simulink model "CascadeControlSim"  (R2022b)
settings: Solver=VariableStepAuto  StartTime=0.0  StopTime=10.0  RelTol=1e-3
values from neighbouring files (symbols this model uses):
  biais_gyr = 1    [Set_Context_CFTE.m]
  Fmax = 0.17*PWM_max + -176.21    (= 121.29)    [Set_Context_CFTE.m]
  Fmin = 0.17*PWM_min + -176.21    (= 2.29)    [Set_Context_CFTE.m]
  Fmoy = 0.17*PWM_moy + -176.21    (= 53.29)    [Set_Context_CFTE.m]
  fr = 0.1    [Set_Context_CFTE.m]
  freq = 0.5    [Set_Context_CFTE.m]
  g = 9.81    [Set_Context_CFTE.m]
  I = 0.07110579    [Set_Context_CFTE.m]
  K1 = 4    [Set_Context_CFTE.m]
  K2 = 128    [Set_Context_CFTE.m]
  Kteta = 20    [Set_Context_CFTE.m]
  l1 = l2    (= 0.363)    [Set_Context_CFTE.m]
  sigma_acc = 0.022    [Set_Context_CFTE.m]
  sigma_gyr = 0.01047    [Set_Context_CFTE.m]
  Tcalibration = 0.5    [Set_Context_CFTE.m]
  Techelon = 4    [Set_Context_CFTE.m]
  theta_max = 0.785398    [Set_Context_CFTE.m]
  theta_ref = -pi()/4    [Set_Context_CFTE.m]
  Ts = 0.08    [Set_Context_CFTE.m]
undefined symbols (not defined in the file or in its folder): DiscIntNeverNeededParam, Rows
libraries: simulink x2, dspsigops x1, dspsrcs4 x1
settings Model: Creator=Hugo  LastModifiedBy=Hugo

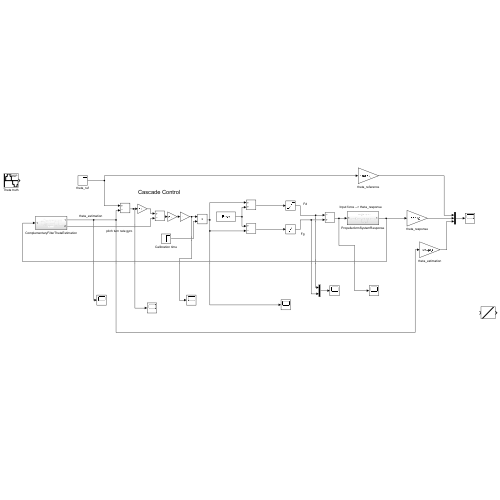
[thumbnail: Simulink's stored preview of the top-level diagram]
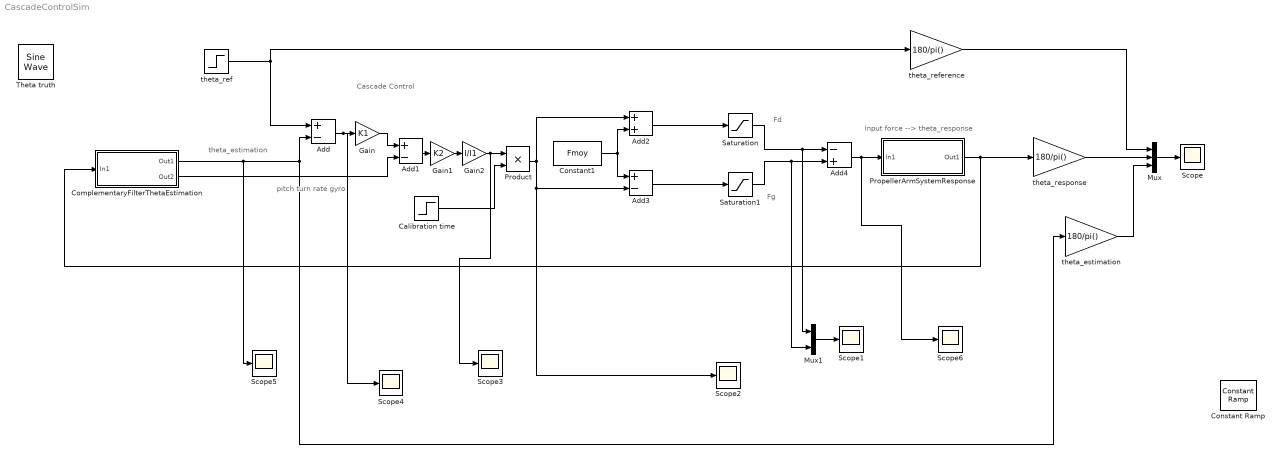
== system CascadeControlSim ==
  note: Cascade Control
  note: Fg
  note: Fd
  note: pitch turn rate gyro
  note: theta_estimation
  note: Input force --> theta_response
  Add : Sum  Inputs=+-
  Add1 : Sum  Inputs=+-
  Add2 : Sum
  Add3 : Sum  Inputs=+-
  Add4 : Sum  Inputs=-+
  Calibration time : Step  Time=Tcalibration  SampleTime=0
  ComplementaryFilterThetaEstimation : Subsystem
  Constant Ramp : dspsigops/Constant Ramp  L=Rows  dim=1  Slope=0.17  dataType=Same as input  isSigned=on  wordLen=16  udDataType=sfix(16)  fracBitsMode=Best precision  numFracBits=15  Offset=-176.21
  Constant1 : Constant  Value=Fmoy
  Gain : Gain  Gain=K1
  Gain1 : Gain  Gain=K2
  Gain2 : Gain  Gain=I/l1
  Mux : Mux  Inputs=3
  Mux1 : Mux  Inputs=2
  Product : Product
  PropellerArmSystemResponse : Subsystem
  Saturation : Saturate  UpperLimit=Fmax  LowerLimit=Fmin
  Saturation1 : Saturate  UpperLimit=Fmax  LowerLimit=Fmin
  Scope{,1..6} (7 alike) : Scope
  Theta truth : dspsrcs4/Sine Wave  Amplitude=theta_max  Frequency=freq  Phase=0  SampleMode=Discrete  OutComplex=Real  CompMethod=Trigonometric fcn  TableSize=Speed  SampleTime=1/1000  SamplesPerFrame=1  ResetState=Restart at time zero  OutputFrames=off  dataType=double  wordLen=16  udDataType=sfix(16)  fracBitsMode=Best precision  numFracBits=15  OutDataTypeStr=double  LastOutDataTypeStr=double
  theta_estimation : Gain  Gain=180/pi()
  theta_ref : Step  Time=Techelon  Before=theta_ref  After=0  SampleTime=0
  theta_reference : Gain  Gain=180/pi()
  theta_response : Gain  Gain=180/pi()
  wires:
  Mux/1 -> Scope/1
  ComplementaryFilterThetaEstimation/1(Out1) -> Scope5/1, theta_estimation/1, Add/2
  theta_ref/1 -> theta_reference/1, Add/1
  Add/1 -> Scope4/1, Gain/1
  Gain/1 -> Add1/1
  ComplementaryFilterThetaEstimation/2(Out2) -> Add1/2
  Add1/1 -> Gain1/1
  Constant1/1 -> Add2/2, Add3/1
  Gain1/1 -> Gain2/1
  Add2/1 -> Saturation/1
  Add3/1 -> Saturation1/1
  Add4/1 -> Scope6/1, PropellerArmSystemResponse/1(In1)
  PropellerArmSystemResponse/1(Out1) -> theta_response/1, ComplementaryFilterThetaEstimation/1(In1)
  Gain2/1 -> Scope3/1, Product/1
  Product/1 -> Add2/1, Scope2/1, Add3/2
  Calibration time/1 -> Product/2
  theta_reference/1 -> Mux/1
  theta_response/1 -> Mux/2
  theta_estimation/1 -> Mux/3
  Saturation1/1 -> Mux1/2, Add4/2
  Saturation/1 -> Add4/1, Mux1/1
  Mux1/1 -> Scope1/1

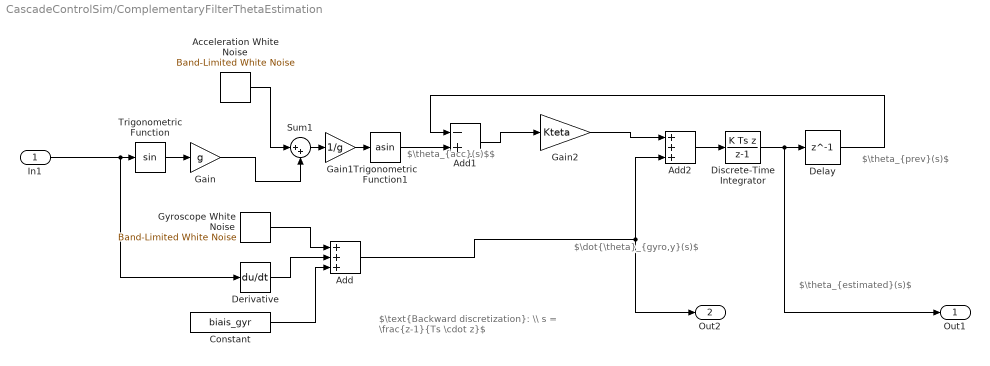
== system CascadeControlSim/ComplementaryFilterThetaEstimation ==
  note: $\theta_{prev}(s)$
  note: $\dot{\theta}_{gyro,y}(s)$
  note: $\text{Backward discretization}: \\ s = \frac{z-1}{Ts \cdot z}$
  note: $\theta_{acc}(s)$$
  note: $\theta_{estimated}(s)$
  In1 : Inport
  " Acceleration White Noise" : simulink/Sources/Band-Limited White Noise  Cov=[sigma_acc]  Ts=Ts  seed=[23341]
  Add : Sum  Inputs=+++
  Add1 : Sum  Inputs=-+
  Add2 : Sum  Inputs=+++
  Constant : Constant  Value=biais_gyr
  Delay : Delay  DelayLength=1  InitialCondition=0
  Derivative : Derivative
  Discrete-Time Integrator : DiscreteIntegrator  IntegratorMethod=Integration: Backward Euler  SampleTime=-1  ICPrevOutput=DiscIntNeverNeededParam  ICPrevScaledInput=DiscIntNeverNeededParam
  Gain : Gain  Gain=g
  Gain1 : Gain  Gain=1/g
  Gain2 : Gain  Gain=Kteta
  Gyroscope White Noise : simulink/Sources/Band-Limited White Noise  Cov=[sigma_gyr]  Ts=Ts  seed=[23341]
  Sum1 : Sum  Inputs=|++
  Trigonometric Function : Trigonometry
  Trigonometric Function1 : Trigonometry  Operator=asin
  Out1 : Outport
  Out2 : Outport  Port=2
  wires:
  Add/1 -> Out2/1, Add2/3
  Derivative/1 -> Add/2
  Delay/1 -> Add1/1
  Trigonometric Function1/1 -> Add1/2
  In1/1 -> Derivative/1, Trigonometric Function/1
  " Acceleration White Noise"/1 -> Sum1/1
  Add2/1 -> Discrete-Time Integrator/1
  Trigonometric Function/1 -> Gain/1
  Sum1/1 -> Gain1/1
  Gyroscope White Noise/1 -> Add/1
  Constant/1 -> Add/3
  Gain1/1 -> Trigonometric Function1/1
  Gain/1 -> Sum1/2
  Add1/1 -> Gain2/1
  Gain2/1 -> Add2/1
  Discrete-Time Integrator/1 -> Out1/1, Delay/1

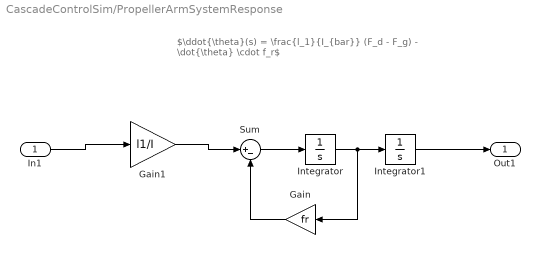
== system CascadeControlSim/PropellerArmSystemResponse ==
  note: $\ddot{\theta}(s) = \frac{l_1}{I_{bar}} (F_d - F_g) - \dot{\theta} \cdot f_r$
  In1 : Inport
  Gain : Gain  Gain=fr
  Gain1 : Gain  Gain=l1/I
  Integrator : Integrator
  Integrator1 : Integrator
  Sum : Sum  Inputs=|+-
  Out1 : Outport
  wires:
  Integrator/1 -> Gain/1, Integrator1/1
  Gain/1 -> Sum/2
  Gain1/1 -> Sum/1
  In1/1 -> Gain1/1
  Sum/1 -> Integrator/1
  Integrator1/1 -> Out1/1
